simulink model "Gas_Calibration"  (R2014a)
settings: Solver=FixedStepDiscrete  StartTime=0.0  StopTime=inf  FixedStep=0.0005  RelTol=1e-3
libraries: ec55xxlib x5
settings Model: Creator=zxj  LastModifiedBy=zxj
settings OptimizationCC: InlineParams=on  InlineInvariantSignals=on  RollThreshold=9  StateBitsets=on  DataBitsets=on  UseTempVars=on  ZeroExternalMemoryAtStartup=off  ZeroInternalMemoryAtStartup=off  EfficientFloat2IntCast=on  OptimizeModelRefInitCode=on  LifeSpan=1
settings DebuggingCC: InheritedTsInSrcMsg=none
settings HardwareCC: ProdLargestAtomicInteger=Long  ProdLargestAtomicFloat=Double  ProdIntDivRoundTo=Zero  ProdEndianess=BigEndian  ProdHWDeviceType=Freescale MPC5500
settings RTWCC: SystemTargetFile=ec55xx.tlc  MakeCommand=make_rtw optimized_fixed_point=1  GenerateMakefile=off  TemplateMakefile=ec55xx_lcc.tmf  PostCodeGenCommand=ec55xx_pst_s2(buildInfo)  Description=Target for EC55XX  GenerateReport=on  ProcessScript=ec55xx_make_rtw_hook  IncludeHyperlinkInReport=on  LaunchReport=on
settings CodeAppCC: IgnoreCustomStorageClasses=off
settings STFCustomTargetCC: ModelReferenceCompliant=off  ConcurrentExecutionCompliant=off  IncludeMdlTerminateFcn=off  GeneratePreprocessorConditionals=Use local settings  CombineOutputUpdateFcns=on  SuppressErrorStatus=on  ERTCustomFileBanners=on  SupportContinuousTime=off  SupportNonInlinedSFcns=off  MATLABClassNameForMDSCustomization=Simulink.SoftwareTarget.ERTCustomization  GRTInterface=off  SystemTargetFile=ec55xx.tlc
settings ERTTargetCC: GenerateSampleERTMain=off  ModelReferenceCompliant=off  IncludeMdlTerminateFcn=off  SuppressErrorStatus=on  GenerateASAP2=on  ERTSrcFileBannerTemplate=ec55xx_code_template.cgt  ERTHdrFileBannerTemplate=ec55xx_code_template.cgt  ERTDataSrcFileTemplate=ec55xx_code_template.cgt  ERTDataHdrFileTemplate=ec55xx_code_template.cgt  ERTCustomFileTemplate=ec55xx_file_process.tlc

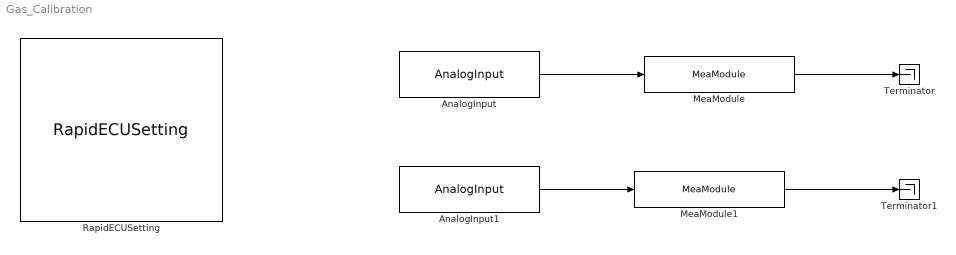
== system Gas_Calibration ==
  AnalogInput : ec55xxlib/RapidECU_U2/02AnalogInput/AnalogInput  channel=54: I_AN15_5V  sampletime=-1
  AnalogInput1 : ec55xxlib/RapidECU_U2/02AnalogInput/AnalogInput  channel=56: I_AN17_5V  sampletime=-1
  MeaModule : ec55xxlib/RapidECU_U2/11Calibration/MeaModule  signal=Gas1
  MeaModule1 : ec55xxlib/RapidECU_U2/11Calibration/MeaModule  signal=Gas2
  RapidECUSetting : ec55xxlib/RapidECU_U2/RapidECUSetting
      link override CAN: bcmt=Extended(29-bit ID)
      link override RTI: rtiperiod=0.0005
  Terminator : Terminator
  Terminator1 : Terminator
  wires:
  AnalogInput/1 -> MeaModule/1
  AnalogInput1/1 -> MeaModule1/1
  MeaModule/1 -> Terminator/1
  MeaModule1/1 -> Terminator1/1
